simulink model "System_composer__model_pre_alpha_V2"  (R2022b)
settings: Solver=VariableStepAuto  StartTime=0.0  StopTime=10.0  RelTol=1e-3
(part 3 of 3)

== system System_composer__model_pre_alpha_V2/Actuate Robot/StopSignalisFalse/F5 Pick Product/F5.6 Activate Gripper ==
  Bus Element In2 : Inport  PortName=New Force value
  Bus Element In1 : Inport  Port=2  PortName=Ready to pick Pick Product
  Bus Element Out2 : Outport  PortName=Current Force
  Bus Element Out1 : Outport  Port=2  PortName=Product Picked

== system System_composer__model_pre_alpha_V2/Actuate Robot/StopSignalisFalse/F6 Translate Product/F6.1 Move ==
  Bus Element In1 : Inport  PortName=Product Picked
  Bus Element Out1 : Outport  PortName=Ready to be Placed

== system System_composer__model_pre_alpha_V2/Actuate Robot/StopSignalisFalse/F7 Place Product/F7.1 Check and Verify force and position of Gripper ==
  Bus Element In1 : Inport  PortName=Corrected Postion
  Bus Element Out1 : Outport  PortName=New Position

== system System_composer__model_pre_alpha_V2/Actuate Robot/StopSignalisFalse/F7 Place Product/F7.2 Lower the Gripper ==
  Bus Element In3 : Inport  PortName=Current Position
  Bus Element In1 : Inport  Port=2  PortName=Ready to be placed
  Bus Element In2 : Inport  Port=3  PortName=New Position
  Bus Element Out1 : Outport  PortName=Gripper Lowered

== system System_composer__model_pre_alpha_V2/Actuate Robot/StopSignalisFalse/F7 Place Product/F7.3 Release the Gripper ==
  Bus Element In1 : Inport  PortName=Gripper Lowered
  Bus Element Out1 : Outport  PortName=Product Released

== system System_composer__model_pre_alpha_V2/Actuate Robot/StopSignalisFalse/F7 Place Product/F7.4 Raise the Gripper ==
  Bus Element In1 : Inport  PortName=Product Released
  Bus Element Out1 : Outport  PortName=Procuct Placed

== system System_composer__model_pre_alpha_V2/Actuate Robot/StopSignalisFalse/F08 Handle Contingencies/Check Pick Position/Around the specified area ==
  Bus Element Out1 : Outport  PortName=Corrected position

== system System_composer__model_pre_alpha_V2/Actuate Robot/StopSignalisFalse/F08 Handle Contingencies/Check Pick Position/Beyond the range ==
